simulink model "MAS_C4_Example4"  (R2021b)
settings: Solver=VariableStepAuto  StartTime=0.0  StopTime=10  RelTol=1e-3
libraries: cstblocks x6
settings Model: Creator=lenovo  LastModifiedBy=lenovo

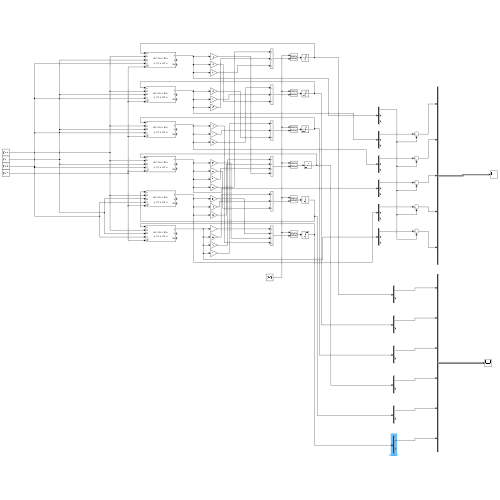
[thumbnail: Simulink's stored preview of the top-level diagram]
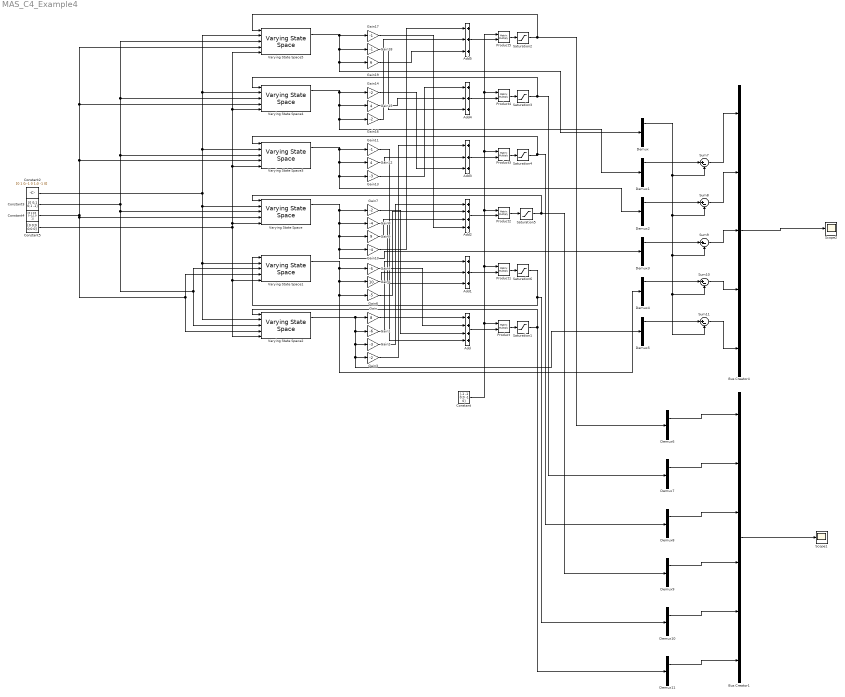
== system MAS_C4_Example4 ==
  Add : Sum  Inputs=++++
  Add{1,3..5} (4 alike) : Sum  Inputs=+++
  Add2 : Sum  Inputs=++++
  Bus Creator1 : BusCreator  Inputs=6
  Bus Creator4 : BusCreator  Inputs=5
  Constant : Constant  Value=[-1 -1 0;0 -1 0]
  Constant2 : Constant  Value=[0 1 0;-1 0 1;0 -1 0]
  Constant3 : Constant  Value=[0 0;1 0;1 -1]
  Constant4 : Constant  Value=[0 1 2;0 0 -1;1 0 1]  VectorParams1D=off
  Constant5 : Constant  Value=[0 0;0 0;0 0]  VectorParams1D=off
  Demux{,1..5} (6 alike) : Demux  Outputs=3
  Demux{6..11} (6 alike) : Demux  Outputs=2
  Gain : Gain  Gain=8
  Gain1 : Gain  Gain=-6
  Gain10 : Gain  Gain=-4
  Gain11 : Gain  Gain=-1
  Gain12 : Gain  Gain=4
  Gain13 : Gain  Gain=-3
  Gain{3,7,14,16} (4 alike) : Gain  Gain=-2
  Gain15 : Gain  Gain=4
  Gain17 : Gain  Gain=-1
  Gain18 : Gain  Gain=-1
  Gain19 : Gain  Gain=6
  Gain2 : Gain  Gain=-3
  Gain4 : Gain  Gain=-5
  Gain5 : Gain  Gain=10
  Gain6 : Gain  Gain=-5
  Gain8 : Gain  Gain=-4
  Gain9 : Gain  Gain=9
  Product{,1..5} (6 alike) : Product  Multiplication=Matrix(*)
  Saturation{1..6} (6 alike) : Saturate  UpperLimit=1  LowerLimit=-1
  Scope1 : Scope
  Scope2 : Scope
  Sum{7..11} (5 alike) : Sum  Inputs=|+-
  Varying State Space : cstblocks/Linear Parameter Varying/Varying State Space  x0=[-2;1;1]  xNames=''  OutputX=on  OutputDX=on
  Varying State Space1 : cstblocks/Linear Parameter Varying/Varying State Space  x0=[2;2;-1]  xNames=''  OutputX=on  OutputDX=on
  Varying State Space2 : cstblocks/Linear Parameter Varying/Varying State Space  x0=[-1;1;2]  xNames=''  OutputX=on  OutputDX=on
  Varying State Space3 : cstblocks/Linear Parameter Varying/Varying State Space  x0=[-1;-1;-2]  xNames=''  OutputX=on  OutputDX=on
  Varying State Space4 : cstblocks/Linear Parameter Varying/Varying State Space  x0=[-3;2;-1]  xNames=''  OutputX=on  OutputDX=on
  Varying State Space5 : cstblocks/Linear Parameter Varying/Varying State Space  x0=[3;-2;-1]  xNames=''  OutputX=on  OutputDX=on
  wires:
  Bus Creator4/1 -> Scope2/1
  Constant2/1 -> Varying State Space3/2, Varying State Space4/2, Varying State Space5/2, Varying State Space2/2, Varying State Space1/2, Varying State Space/2
  Constant3/1 -> Varying State Space3/3, Varying State Space4/3, Varying State Space5/3, Varying State Space2/3, Varying State Space1/3, Varying State Space/3
  Constant4/1 -> Varying State Space3/4, Varying State Space4/4, Varying State Space5/4, Varying State Space2/4, Varying State Space1/4, Varying State Space/4
  Constant5/1 -> Varying State Space/5, Varying State Space5/5, Varying State Space4/5, Varying State Space3/5, Varying State Space2/5, Varying State Space1/5
  Demux3/1 -> Sum9/1
  Demux4/1 -> Sum10/1
  Demux5/1 -> Sum11/1
  Demux2/1 -> Sum8/1
  Demux1/1 -> Sum7/1
  Demux/1 -> Sum8/2, Sum11/2, Sum10/2, Sum9/2, Sum7/2
  Sum9/1 -> Bus Creator4/3
  Sum8/1 -> Bus Creator4/2
  Sum7/1 -> Bus Creator4/1
  Sum11/1 -> Bus Creator4/5
  Sum10/1 -> Bus Creator4/4
  Varying State Space2/1 -> Demux5/1, Gain3/1, Gain2/1, Gain1/1, Gain/1
  Varying State Space1/1 -> Demux4/1, Gain6/1, Gain5/1, Gain4/1
  Varying State Space/1 -> Demux3/1, Gain10/1, Gain9/1, Gain8/1, Gain7/1
  Varying State Space3/1 -> Demux2/1, Gain13/1, Gain12/1, Gain11/1
  Varying State Space4/1 -> Gain14/1, Demux1/1, Gain16/1, Gain15/1
  Varying State Space5/1 -> Demux/1, Gain19/1, Gain18/1, Gain17/1
  Gain/1 -> Add/1
  Gain4/1 -> Add/2
  Gain7/1 -> Add/3
  Gain11/1 -> Add/4
  Gain1/1 -> Add1/1
  Gain5/1 -> Add1/2
  Gain8/1 -> Add1/3
  Gain2/1 -> Add2/1
  Gain6/1 -> Add2/2
  Gain9/1 -> Add2/3
  Gain17/1 -> Add2/4
  Gain3/1 -> Add3/1
  Gain12/1 -> Add3/2
  Gain14/1 -> Add3/3
  Gain13/1 -> Add4/1
  Gain15/1 -> Add4/2
  Gain18/1 -> Add4/3
  Gain19/1 -> Add5/3
  Gain16/1 -> Add5/2
  Gain10/1 -> Add5/1
  Add5/1 -> Product5/2
  Add4/1 -> Product4/2
  Add3/1 -> Product3/2
  Add2/1 -> Product2/2
  Add1/1 -> Product1/2
  Add/1 -> Product/2
  Constant/1 -> Product5/1, Product4/1, Product3/1, Product2/1, Product1/1, Product/1
  Saturation2/1 -> Demux6/1, Varying State Space5/1
  Saturation3/1 -> Demux7/1, Varying State Space4/1
  Saturation4/1 -> Demux8/1, Varying State Space3/1
  Saturation5/1 -> Demux9/1, Varying State Space/1
  Saturation6/1 -> Demux10/1, Varying State Space1/1
  Saturation1/1 -> Varying State Space2/1, Demux11/1
  Product/1 -> Saturation1/1
  Product5/1 -> Saturation2/1
  Product4/1 -> Saturation3/1
  Product3/1 -> Saturation4/1
  Product2/1 -> Saturation5/1
  Product1/1 -> Saturation6/1
  Bus Creator1/1 -> Scope1/1
  Demux6/1 -> Bus Creator1/1
  Demux7/1 -> Bus Creator1/2
  Demux8/1 -> Bus Creator1/3
  Demux9/1 -> Bus Creator1/4
  Demux10/1 -> Bus Creator1/5
  Demux11/1 -> Bus Creator1/6
